simulink model "MecanumPose"  (R2019b)
settings: Solver=FixedStepAuto  StartTime=0.0  StopTime=inf  FixedStep=0.01  RelTol=1e-3
InitFcn:
  | mecanum_init
values from neighbouring files (symbols this model uses):
  J3 = (1/r)*[1 1 a+b ... (first row only)    [mecanum_init.m]
undefined symbols (not defined in the file or in its folder): canChannel, DiscIntNeverNeededParam
libraries: etargetslib x4, canmsglib x4, canlib x2, aerolibutil x1
settings Model: Creator=giull  LastModifiedBy=giull
settings OptimizationCC: EnhancedBackFolding=on  PassReuseOutputArgsAs=Individual arguments  ZeroExternalMemoryAtStartup=off  ZeroInternalMemoryAtStartup=off  MaxStackSize=64  OptimizeBlockOrder=speed  DifferentSizesBufferReuse=on  OptimizationCustomize=off  EfficientTunableParamExpr=on
settings DebuggingCC: ParameterTunabilityLossMsg=error
settings HardwareCC: ProdBitPerPointer=32  ProdBitPerSizeT=32  ProdBitPerPtrDiffT=32  ProdLargestAtomicFloat=None  ProdIntDivRoundTo=Undefined  ProdEndianess=Unspecified  ProdWordSize=32  ProdHWDeviceType=Generic->Unspecified (assume 32-bit Generic)
settings SFSimCC: MATLABDynamicMemAlloc=off
settings RTWCC: SystemTargetFile=ert.tlc  HardwareBoard=Robot Operating System (ROS)  TLCOptions="-aInlineSetEventsForThisBaseRateFcn=TLC_FALSE -aSuppressMultiTaskScheduler=TLC_FALSE  -aRateBasedStepFcn=0"  TemplateMakefile=ert_default_tmf  GenerateReport=on  Toolchain=Catkin  IncludeHyperlinkInReport=on  LaunchReport=on  TargetLang=C++  GenerateTraceInfo=on  GenerateTraceReport=on  GenerateTraceReportSl=on  GenerateTraceReportSf=on  GenerateTraceReportEml=on
settings CodeAppCC: ForceParamTrailComments=on  IgnoreCustomStorageClasses=off  OperatorAnnotations=on  SimulinkDataObjDesc=on  SFDataObjDesc=on  InsertBlockDesc=on

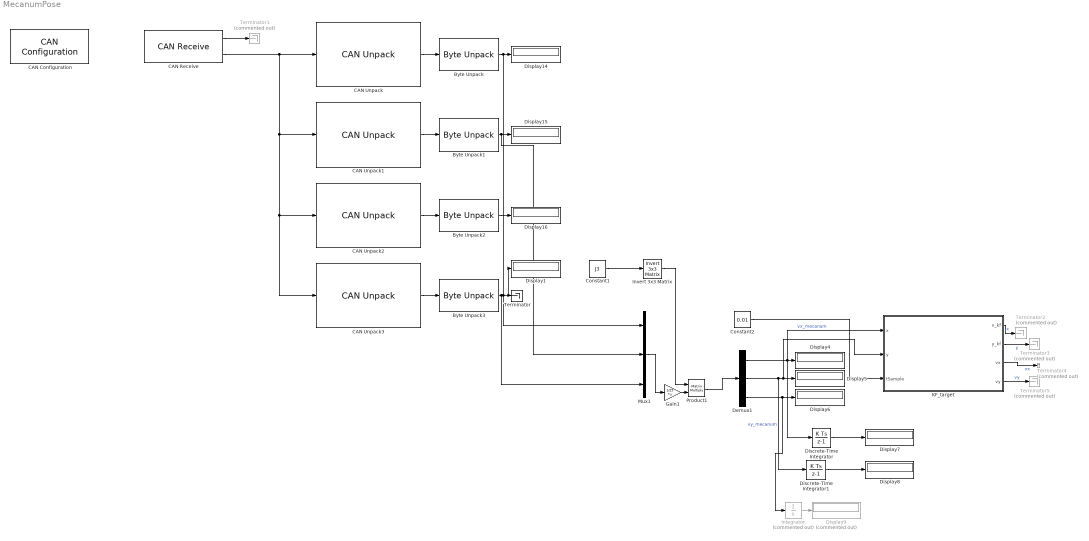
== system MecanumPose ==
  Byte Unpack{,1..3} (4 alike) : etargetslib/Byte Unpack  dimensions={[1]}  datatypes={'int16'}  byteAlign=1
      settings: SourceProductName=MATLAB Coder
  CAN Configuration : canlib/CAN Configuration  BlockHandle=6.0006  Device=PEAK-System PCAN-USB (PCAN_USBBUS1)  DeviceMenu=PEAK-System PCAN-USB (PCAN_USBBUS1)  ObjConstructor=canChannel('PEAK-System', 'PCAN_USBBUS1')  BusSpeed=500000  EnableBitParameters=off  AckMode=Normal
      settings: SourceProductName=Vehicle Network Toolbox  SourceProductBaseCode=VN
  CAN Receive : canlib/CAN Receive  BlockHandle=7.0006  Device=PEAK-System PCAN-USB (PCAN_USBBUS1)  DeviceMenu=PEAK-System PCAN-USB (PCAN_USBBUS1)  ObjConstructor=canChannel('PEAK-System', 'PCAN_USBBUS1')  EnableStandardIDsFilter=off  StdIDsCombo=Allow all  StandardIDs=275  EnableExtendedIDsFilter=off  ExtIDsCombo=Allow all  ExtendedIDs=275  SampleTime=0.01  MsgsPerTimestep=all  InternalFilterUpdateStatus=on  BusOutput=on
      settings: SourceProductName=Vehicle Network Toolbox  SourceProductBaseCode=VN
  CAN Unpack : canmsglib/CAN Unpack  MsgList=(none)  MsgName=CAN Msg  MsgIDType=Standard (11-bit identifier)  MsgIdentifier=275  MsgLength=2  SignalInfo={ 'Signal1', '0', '64', 'LE', 'signed', 'Standard', '0', '1', '0', '-Inf', 'Inf' }  IDPort=off  TimestampPort=off  ErrorPort=off  RemotePort=off  LengthPort=off  StatusPort=off  ApplyMinMax=off
      settings: SourceProductName=Vehicle Network Toolbox  SourceProductBaseCode=VN  DataFormat=raw data
  CAN Unpack1 : canmsglib/CAN Unpack  MsgList=(none)  MsgName=CAN Msg  MsgIDType=Standard (11-bit identifier)  MsgIdentifier=259  MsgLength=2  SignalInfo={ 'Signal1', '0', '64', 'LE', 'signed', 'Standard', '0', '1', '0', '-Inf', 'Inf' }  IDPort=off  TimestampPort=off  ErrorPort=off  RemotePort=off  LengthPort=off  StatusPort=off  ApplyMinMax=off
      settings: SourceProductName=Vehicle Network Toolbox  SourceProductBaseCode=VN  DataFormat=raw data
  CAN Unpack2 : canmsglib/CAN Unpack  MsgList=(none)  MsgName=CAN Msg  MsgIDType=Standard (11-bit identifier)  MsgIdentifier=291  MsgLength=2  SignalInfo={ 'Signal1', '0', '64', 'LE', 'signed', 'Standard', '0', '1', '0', '-Inf', 'Inf' }  IDPort=off  TimestampPort=off  ErrorPort=off  RemotePort=off  LengthPort=off  StatusPort=off  ApplyMinMax=off
      settings: SourceProductName=Vehicle Network Toolbox  SourceProductBaseCode=VN  DataFormat=raw data
  CAN Unpack3 : canmsglib/CAN Unpack  MsgList=(none)  MsgName=CAN Msg  MsgIDType=Standard (11-bit identifier)  MsgIdentifier=307  MsgLength=2  SignalInfo={ 'Signal1', '0', '64', 'LE', 'signed', 'Standard', '0', '1', '0', '-Inf', 'Inf' }  IDPort=off  TimestampPort=off  ErrorPort=off  RemotePort=off  LengthPort=off  StatusPort=off  ApplyMinMax=off
      settings: SourceProductName=Vehicle Network Toolbox  SourceProductBaseCode=VN  DataFormat=raw data
  Constant1 : Constant  Value=J3
  Constant2 : Constant  Value=0.01
  Demux1 : Demux  Outputs=3
  Discrete-Time Integrator : DiscreteIntegrator  SampleTime=-1  ICPrevOutput=DiscIntNeverNeededParam  ICPrevScaledInput=DiscIntNeverNeededParam
  Discrete-Time Integrator1 : DiscreteIntegrator  SampleTime=-1  ICPrevOutput=DiscIntNeverNeededParam  ICPrevScaledInput=DiscIntNeverNeededParam
  Display{1,4..8,14..16} (9 alike) : Display
  Display9 : Display  Commented=on
  Gain1 : Gain  Gain=1/25  Multiplication=Matrix(K*u)
  Integrator : Integrator  Commented=on
  Invert 3x3 Matrix : aerolibutil/Invert  3x3 Matrix
  KF_target : MATLAB Function  TreatAsAtomicUnit=on
  Mux1 : Mux  Inputs=3
  Product1 : Product  Multiplication=Matrix(*)
  Terminator : Terminator
  Terminator{1..5} (5 alike) : Terminator  Commented=on
  wires:
  Constant1/1 -> Invert 3x3 Matrix/1
  Product1/1 -> Demux1/1
  Demux1/1 -> Discrete-Time Integrator/1, KF_target/1(x), Display4/1  "vx_mecanum"
  Demux1/2 -> Discrete-Time Integrator1/1, KF_target/2(y), Display5/1  "vy_mecanum"
  Demux1/3 -> Integrator/1, Display6/1
  Invert 3x3 Matrix/1 -> Product1/1
  Integrator/1 -> Display9/1
  Discrete-Time Integrator1/1 -> Display8/1
  Discrete-Time Integrator/1 -> Display7/1
  Byte Unpack/1 -> Mux1/1, Display14/1
  Byte Unpack1/1 -> Mux1/2, Display15/1
  Byte Unpack3/1 -> Mux1/3, Display1/1, Terminator/1
  CAN Receive/1 -> Terminator1/1
  CAN Receive/2 -> CAN Unpack3/1, CAN Unpack2/1, CAN Unpack1/1, CAN Unpack/1
  CAN Unpack/1 -> Byte Unpack/1
  CAN Unpack2/1 -> Byte Unpack2/1
  CAN Unpack1/1 -> Byte Unpack1/1
  CAN Unpack3/1 -> Byte Unpack3/1
  Byte Unpack2/1 -> Display16/1
  Constant2/1 -> KF_target/3(tSample)
  Mux1/1 -> Gain1/1
  Gain1/1 -> Product1/2
  KF_target/1(x_kf) -> Terminator2/1  "x"
  KF_target/2(y_kf) -> Terminator3/1  "y"
  KF_target/3(vx) -> Terminator4/1  "vx"
  KF_target/4(vy) -> Terminator5/1  "vy"

== matlab function MecanumPose/KF_target ==
  settings: updateMethod=DISCRETE
  data: x input; y input; x_kf output; tSample input; y_kf output; vx output; vy output
function [x_kf,y_kf,vx,vy]   = fcn(x,y,tSample)

persistent x_dach P Q R C I A_d firstRun A

if isempty(firstRun)
    
  firstRun = 1;
  
     I=eye(6);

     A = [0 0 1 0 0 0;
          0 0 0 1 0 0;
          0 0 0 0 1 0;
          0 0 0 0 0 1;
          0 0 0 0 0 0;
          0 0 0 0 0 0];
      
     A_d = expm(A*tSample);
       
    C=[0 0 1 0 0 0
       0 0 0 1 0 0];

    Q=0.001*I;

    R=1*eye(2);

    P = 0.1*I;

    x_dach = [0 0 0 0 0 0]'; % Startwerte phi theta psi

end


%% Kalman Filter


xp = A_d*x_dach;

Pp = A_d*P*A_d' + Q;    

K = Pp*C'*inv(C*Pp*C' + R);

x_dach = xp + K*([x y]' - C*xp);

P = Pp - K*C*Pp;

x_kf=x_dach(1);
y_kf=x_dach(2);
vx = x_dach(3);
vy = x_dach(4);
end
